simulink model "Mission_TJ1000_ResponseTest"  (R2019a)
settings: Solver=FixedStepAuto  StartTime=0.0  StopTime=170  FixedStep=0.2  RelTol=1e-3
settings Model: Creator=anton  LastModifiedBy=anton

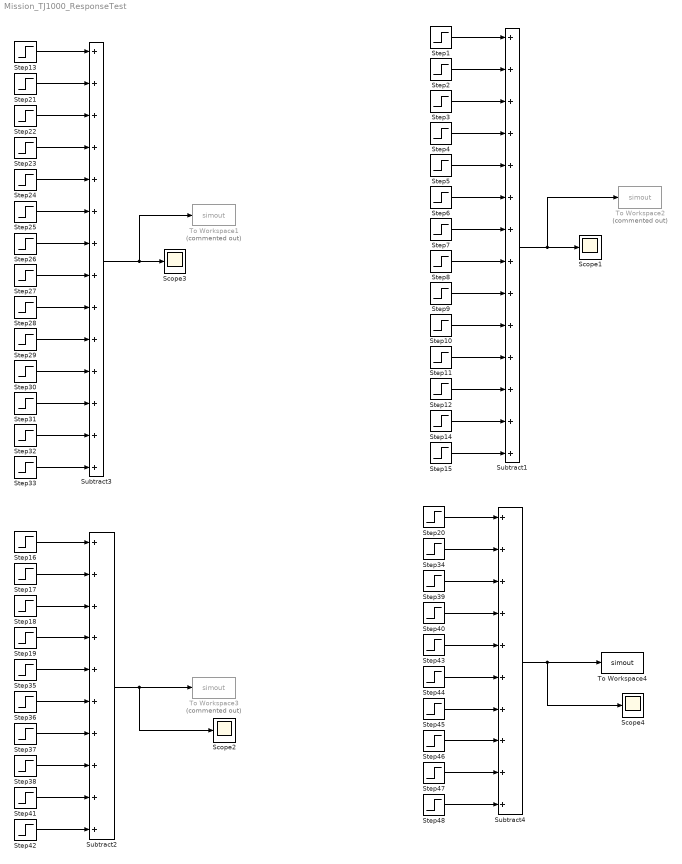
== system Mission_TJ1000_ResponseTest ==
  Scope{1..4} (4 alike) : Scope
  Step1 : Step  Time=153  After=2000  SampleTime=0
  Step10 : Step  Time=243  After=-500  SampleTime=0
  Step11 : Step  Time=253  After=-500  SampleTime=0
  Step12 : Step  Time=263  After=-500  SampleTime=0
  Step13 : Step  Time=3  After=2000  SampleTime=0
  Step14 : Step  Time=273  After=2700  SampleTime=0
  Step15 : Step  Time=283  After=-2700  SampleTime=0
  Step16 : Step  Time=10  Before=1500  After=2000  SampleTime=0
  Step17 : Step  Time=20  After=500  SampleTime=0
  Step18 : Step  Time=30  After=500  SampleTime=0
  Step19 : Step  Time=40  After=500  SampleTime=0
  Step2 : Step  Time=163  After=500  SampleTime=0
  Step20 : Step  Time=70  Before=1500  After=2000  SampleTime=0
  Step21 : Step  Time=13  After=500  SampleTime=0
  Step22 : Step  Time=23  After=500  SampleTime=0
  Step23 : Step  Time=33  After=500  SampleTime=0
  Step24 : Step  Time=43  After=300  SampleTime=0
  Step25 : Step  Time=53  After=200  SampleTime=0
  Step26 : Step  Time=63  After=-200  SampleTime=0
  Step27 : Step  Time=73  After=-300  SampleTime=0
  Step28 : Step  Time=83  After=-500  SampleTime=0
  Step29 : Step  Time=93  After=-500  SampleTime=0
  Step3 : Step  Time=173  After=500  SampleTime=0
  Step30 : Step  Time=103  After=-500  SampleTime=0
  Step31 : Step  Time=113  After=-500  SampleTime=0
  Step32 : Step  Time=123  After=2700  SampleTime=0
  Step33 : Step  Time=133  After=-2700  SampleTime=0
  Step34 : Step  Time=80  After=500  SampleTime=0
  Step35 : Step  Time=50  After=-500  SampleTime=0
  Step36 : Step  Time=60  After=-500  SampleTime=0
  Step37 : Step  Time=70  After=-500  SampleTime=0
  Step38 : Step  Time=80  After=-500  SampleTime=0
  Step39 : Step  Time=90  After=500  SampleTime=0
  Step4 : Step  Time=183  After=500  SampleTime=0
  Step40 : Step  Time=100  After=500  SampleTime=0
  Step41 : Step  Time=90  After=2000  SampleTime=0
  Step42 : Step  Time=100  After=-2000  SampleTime=0
  Step43 : Step  Time=110  After=-500  SampleTime=0
  Step44 : Step  Time=120  After=-500  SampleTime=0
  Step45 : Step  Time=130  After=-500  SampleTime=0
  Step46 : Step  Time=140  After=-500  SampleTime=0
  Step47 : Step  Time=150  After=2000  SampleTime=0
  Step48 : Step  Time=160  After=-2000  SampleTime=0
  Step5 : Step  Time=193  After=300  SampleTime=0
  Step6 : Step  Time=203  After=200  SampleTime=0
  Step7 : Step  Time=213  After=-200  SampleTime=0
  Step8 : Step  Time=223  After=-300  SampleTime=0
  Step9 : Step  Time=233  After=-500  SampleTime=0
  Subtract1 : Sum  Inputs=++++++++++++++
  Subtract2 : Sum  Inputs=++++++++++
  Subtract3 : Sum  Inputs=++++++++++++++
  Subtract4 : Sum  Inputs=++++++++++
  To Workspace1 : ToWorkspace  Commented=on  VariableName=simout  SaveFormat=Timeseries  SampleTime=-1
  To Workspace2 : ToWorkspace  Commented=on  VariableName=simout  SaveFormat=Timeseries  SampleTime=-1
  To Workspace3 : ToWorkspace  Commented=on  VariableName=simout  SaveFormat=Timeseries  SampleTime=-1
  To Workspace4 : ToWorkspace  VariableName=simout  SaveFormat=Timeseries  SampleTime=-1
  wires:
  Step29/1 -> Subtract3/10
  Step28/1 -> Subtract3/9
  Step27/1 -> Subtract3/8
  Step26/1 -> Subtract3/7
  Step25/1 -> Subtract3/6
  Step24/1 -> Subtract3/5
  Step23/1 -> Subtract3/4
  Step22/1 -> Subtract3/3
  Step21/1 -> Subtract3/2
  Step13/1 -> Subtract3/1
  Subtract3/1 -> To Workspace1/1, Scope3/1
  Step30/1 -> Subtract3/11
  Step31/1 -> Subtract3/12
  Step32/1 -> Subtract3/13
  Step33/1 -> Subtract3/14
  Step15/1 -> Subtract1/14
  Step14/1 -> Subtract1/13
  Step12/1 -> Subtract1/12
  Step11/1 -> Subtract1/11
  Subtract1/1 -> To Workspace2/1, Scope1/1
  Step1/1 -> Subtract1/1
  Step2/1 -> Subtract1/2
  Step3/1 -> Subtract1/3
  Step4/1 -> Subtract1/4
  Step5/1 -> Subtract1/5
  Step6/1 -> Subtract1/6
  Step7/1 -> Subtract1/7
  Step8/1 -> Subtract1/8
  Step9/1 -> Subtract1/9
  Step10/1 -> Subtract1/10
  Step42/1 -> Subtract2/10
  Step41/1 -> Subtract2/9
  Subtract2/1 -> Scope2/1, To Workspace3/1
  Step16/1 -> Subtract2/1
  Step17/1 -> Subtract2/2
  Step18/1 -> Subtract2/3
  Step19/1 -> Subtract2/4
  Step35/1 -> Subtract2/5
  Step36/1 -> Subtract2/6
  Step37/1 -> Subtract2/7
  Step38/1 -> Subtract2/8
  Step46/1 -> Subtract4/8
  Step45/1 -> Subtract4/7
  Step44/1 -> Subtract4/6
  Step43/1 -> Subtract4/5
  Step40/1 -> Subtract4/4
  Step39/1 -> Subtract4/3
  Step34/1 -> Subtract4/2
  Step20/1 -> Subtract4/1
  Subtract4/1 -> To Workspace4/1, Scope4/1
  Step47/1 -> Subtract4/9
  Step48/1 -> Subtract4/10
